simulink model "untitled"  (R2019b)
settings: Solver=VariableStepAuto  StartTime=0.0  StopTime=10.0  RelTol=1e-3
StartFcn:
  | init.m
values from neighbouring files (symbols this model uses):
  g = 9.8    [init.m]
  l1 = 0.5    [init.m]
  l2 = 0.3    [init.m]
  m1 = 4.6    [init.m]
  m2 = 2.3    [init.m]
settings Model: Creator=xgge2  LastModifiedBy=xgge2

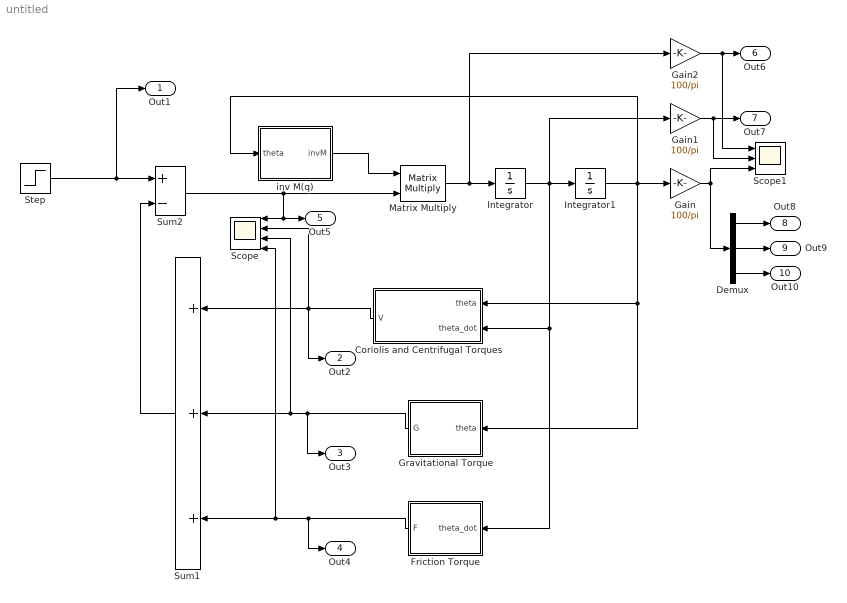
== system untitled ==
  "Coriolis and Centrifugal Torques " : MATLAB Function  TreatAsAtomicUnit=on
  Demux : Demux  Outputs=3
  Friction Torque : MATLAB Function  TreatAsAtomicUnit=on
  Gain : Gain  Gain=100/pi
  Gain1 : Gain  Gain=100/pi
  Gain2 : Gain  Gain=100/pi
  Gravitational Torque : MATLAB Function  TreatAsAtomicUnit=on
  Integrator : Integrator
  Integrator1 : Integrator  InitialCondition=[0 0 0]
  Matrix Multiply : Product  Multiplication=Matrix(*)
  Scope : Scope  NumInputPorts=4
  Scope1 : Scope  NumInputPorts=3
  Step : Step  Before=[0; 0; 0]  After=[0; 0; 0]  SampleTime=0  VectorParams1D=off
  Sum1 : Sum  Inputs=+++
  Sum2 : Sum  Inputs=+-
  inv M(q) : MATLAB Function  TreatAsAtomicUnit=on
  Out1 : Outport  SignalName=tau
  Out2 : Outport  Port=2  SignalName=V
  Out3 : Outport  Port=3  SignalName=G
  Out4 : Outport  Port=4  SignalName=F
  Out5 : Outport  Port=5  SignalName=Result Torque
  Out6 : Outport  Port=6  SignalName=theta_ddot
  Out7 : Outport  Port=7  SignalName=theta_dot
  Out8 : Outport  Port=8  SignalName=theta1
  Out9 : Outport  Port=9  SignalName=theta2
  Out10 : Outport  Port=10  SignalName=theta3
  wires:
  Step/1 -> Out1/1, Sum2/1
  Friction Torque/1(F) -> Scope/4, Sum1/3, Out4/1
  Gravitational Torque/1(G) -> Out3/1, Scope/3, Sum1/2
  "Coriolis and Centrifugal Torques "/1(V) -> Scope/2, Out2/1, Sum1/1
  Sum2/1 -> Matrix Multiply/2, Scope/1, Out5/1
  Sum1/1 -> Sum2/2
  Matrix Multiply/1 -> Gain2/1, Integrator/1
  Integrator/1 -> Friction Torque/1(theta_dot), "Coriolis and Centrifugal Torques "/2(theta_dot), Gain1/1, Integrator1/1
  inv M(q)/1(invM) -> Matrix Multiply/1
  Integrator1/1 -> "Coriolis and Centrifugal Torques "/1(theta), Gravitational Torque/1(theta), Gain/1, inv M(q)/1(theta)
  Gain/1 -> Scope1/3, Demux/1
  Gain2/1 -> Scope1/1, Out6/1
  Gain1/1 -> Scope1/2, Out7/1
  Demux/1 -> Out8/1
  Demux/2 -> Out9/1
  Demux/3 -> Out10/1

== matlab function untitled/Gravitational Torque ==
  data: theta input size=[3,1]; G output size=[3,1]; m1 parameter; m2 parameter; l1 parameter; l2 parameter; g parameter
function G  = fcn(theta, m1, m2, l1, l2, g)
    G = zeros([3,1]);
    G(1) = m2*l2*g*cos(theta(1)+theta(2))+(m1+m2)*l1*g*cos(theta(1));
    G(2) = m2*l2*g*cos(theta(1)+theta(2));
    G(3) = 0;

== matlab function untitled/Coriolis and Centrifugal Torques  ==
  data: theta input size=[3,1]; V output size=[3,1]; theta_dot input size=[3,1]; m2 parameter; l1 parameter; l2 parameter
function V  = fcn(theta,theta_dot,m2, l1, l2)
    V = zeros([3,1]);
    V(1) = -m2*l1*l2*sin(theta(2))*theta_dot(2)^2 - 2*m2*l1*l2*sin(theta(2))*theta_dot(1)*theta_dot(2);
    V(2) = m2*l1*l2*sin(theta(2))*theta_dot(1)^2;
    V(3) = 0;

== matlab function untitled/Friction Torque ==
  data: theta_dot input size=[3,1]; F output size=[3,1]; v parameter
function F = fcn(theta_dot, v)
    F = zeros([3,1]);
    F(1) = v*theta_dot(1);
    F(2) = v*theta_dot(2);
    F(3) = 0;

== matlab function untitled/inv M(q) ==
  data: theta input size=[3,1]; invM output size=[3,3]; m1 parameter; m2 parameter; l1 parameter; l2 parameter
function invM  = fnc(theta, m1, m2, l1, l2)
    M = zeros([3,3]);
    M(1,1) = m2*l2^2 + 2*m2*l1*l2*cos(theta(2))+(l1^2)*(m1+m2);
    M(1,2) = m2*l2^2 + m2*l1*l2*cos(theta(2));
    M(2,1) = m2*l2^2 + m2*l1*l2*cos(theta(2));
    M(2,2) = m2*l2^2;
    invM = inverse(M);
